simulink model "Propagator"  (R2018a)
settings: Solver=ode4  StartTime=jd_start  StopTime=jd_end  FixedStep=3600  MaxStep=stepsize  RelTol=1e-9  AbsTol=1e-12  EnableMultiTasking=on
values from neighbouring files (symbols this model uses):
  state_ast_initial = [xin; yin; zin; vxin; vyin; vzin]    [driverScript.m]
  state_sat_initial = [xin2; yin2; zin2; vxin2; vyin2; vzin2]    [driverScript.m]
settings Model: Creator=Hridu  LastModifiedBy=Hridu
settings SolverCC: AutoScaleAbsTol=off
settings OptimizationCC: LifeSpan=inf
settings DebuggingCC: SFUnexpectedBacktrackingDiag=warning  SFNoUnconditionalDefaultTransitionDiag=warning  SFExecutionAtInitializationDiag=none
settings CodeAppCC: StateflowObjectComments=on
settings GRTTargetCC: TargetLangStandard=C89/C90 (ANSI)  GeneratePreprocessorConditionals=Disable all
settings ConfigComp: CovMetricSettings=dw  CovHtmlReporting=on  CovSaveCumulativeToWorkspaceVar=on  CovSaveSingleToWorkspaceVar=on  CovExternalEMLEnable=off

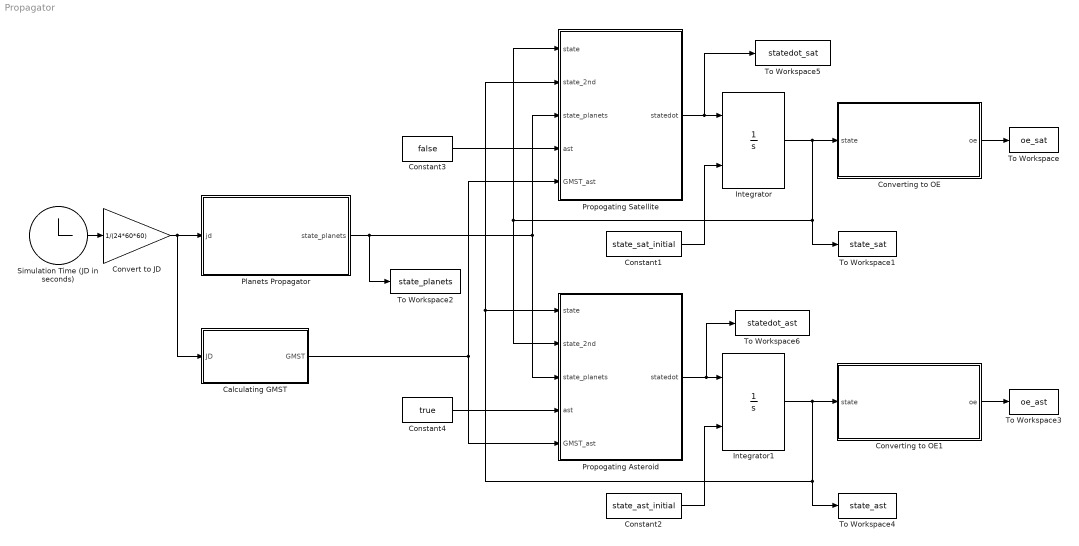
== system Propagator ==
  Calculating GMST : MATLAB Function  TreatAsAtomicUnit=on
  Constant1 : Constant  Value=state_sat_initial
  Constant2 : Constant  Value=state_ast_initial
  Constant3 : Constant  Value=false
  Constant4 : Constant  Value=true
  Convert to JD : Gain  Gain=1/(24*60*60)
  Converting to OE : MATLAB Function  TreatAsAtomicUnit=on
  Converting to OE1 : MATLAB Function  TreatAsAtomicUnit=on
  Integrator : Integrator  InitialConditionSource=external
  Integrator1 : Integrator  InitialConditionSource=external
  Planets Propagator : MATLAB Function  TreatAsAtomicUnit=on
  Propogating Asteroid : MATLAB Function  TreatAsAtomicUnit=on
  Propogating Satellite : MATLAB Function  TreatAsAtomicUnit=on
  Simulation Time (JD in seconds) : Clock
  To Workspace : ToWorkspace  VariableName=oe_sat  SampleTime=-1
  To Workspace1 : ToWorkspace  VariableName=state_sat  SampleTime=-1
  To Workspace2 : ToWorkspace  VariableName=state_planets  SampleTime=-1
  To Workspace3 : ToWorkspace  VariableName=oe_ast  SampleTime=-1
  To Workspace4 : ToWorkspace  VariableName=state_ast  SampleTime=-1
  To Workspace5 : ToWorkspace  VariableName=statedot_sat  SampleTime=-1
  To Workspace6 : ToWorkspace  VariableName=statedot_ast  SampleTime=-1
  wires:
  Propogating Satellite/1(statedot) -> To Workspace5/1, Integrator/1
  Constant1/1 -> Integrator/2
  Converting to OE/1(oe) -> To Workspace/1
  Simulation Time (JD in seconds)/1 -> Convert to JD/1
  Planets Propagator/1(state_planets) -> To Workspace2/1, Propogating Asteroid/3(state_planets), Propogating Satellite/3(state_planets)
  Integrator/1 -> Propogating Asteroid/2(state_2nd), Propogating Satellite/1(state), To Workspace1/1, Converting to OE/1(state)
  Propogating Asteroid/1(statedot) -> To Workspace6/1, Integrator1/1
  Constant2/1 -> Integrator1/2
  Converting to OE1/1(oe) -> To Workspace3/1
  Integrator1/1 -> Converting to OE1/1(state), Propogating Asteroid/1(state), Propogating Satellite/2(state_2nd), To Workspace4/1
  Constant3/1 -> Propogating Satellite/4(ast)
  Constant4/1 -> Propogating Asteroid/4(ast)
  Calculating GMST/1(GMST) -> Propogating Asteroid/5(GMST_ast), Propogating Satellite/5(GMST_ast)
  Convert to JD/1 -> Calculating GMST/1(JD), Planets Propagator/1(jd)

== matlab function Propagator/Converting to OE ==
  data: state input; oe output
function oe = IJKtoOrbitalElements(state)

oe = zeros(6, 1);

% Position and Velocity
rECI = state(1:3);
vECI = state(4:6);

% Specific Angular Momentum
GM_Earth = 3.986e5;
h = cross(rECI, vECI);
W = h./norm(h);

% Inclination
i = atan2(norm(W(1:2)), W(3));

% Right Ascension of the Ascending Node
Omega = atan2(W(1),-W(2));
if Omega < 0
    Omega = Omega + 2*pi;
end

% Semi-Major Axis
a = (2/norm(rECI) - norm(vECI)^2/GM_Earth)^-1;

% Eccentricity
p = norm(h)^2/GM_Earth;
e = sqrt(1 - p/a);

% True Anomaly
n = sqrt(GM_Earth/a^3);
E = atan2((dot(rECI, vECI)/(n*a^2)), (1 - norm(rECI)/a));
if E < 0
    E = E + 2*pi;
end

nu = atan2(a*sqrt(1-e^2)*sin(E),a*(cos(E)-e));
if nu < 0
    nu = nu + 2*pi;
end

% Argument of Periapsis
u = atan2((rECI(3)/sin(i)), (rECI(1)*cos(Omega) + rECI(2)*sin(Omega)));
if u < 0
    u = u + 2*pi;
end

omega = u - nu;
if omega < 0
    omega = omega + 2*pi;
end

oe(1) = a;
oe(2) = e;
oe(3) = i;
oe(4) = Omega;
oe(5) = omega;
oe(6) = nu;

end

== matlab function Propagator/Propogating Satellite ==
  data: state input; state_2nd input; statedot output; state_planets input; ast input; GMST_ast input
function statedot = f(state, state_2nd, state_planets, ast, GMST_ast)

X = load('constants.mat');
statedot = zeros(6, 1);

% Solar Radiation Pressure
if ast == false
    f_srp = accelSRP(state, X.state_sun, state_2nd, X.R_ast,...
        X.Csrp_sat, X.Msrp_sat, X.Asrp_sat, X.Psrp);
else
    f_srp = accelSRP(state, X.state_sun, state_2nd, 0,...
        X.Csrp_ast, X.Msrp_ast, X.Asrp_ast, X.Psrp);
end

% Drag
%f_drag = accelDrag(state);

% Asteroid Gravity
if ast == false
    f_2nd = accelHarmonic(state, state_2nd, X.GM_ast, X.R_ast, GMST_ast);
else
    f_2nd = accelPointMass(state, state_2nd, X.GM_sat);
end

% Sun Gravity
f_sun = X.GM_Sun*state(1:3)/(norm(state(1:3))^3);

% Planets Gravity
f_planets = zeros(3, 1);
for planetid = 1:9
    f_planets = f_planets + accelPointMass(state, state_planets(planetid, :)', X.GM_Planets(planetid));
end

% Calculating StateDot
statedot(1:3) = state(4:6);
statedot(4:6) = -1*(f_2nd + f_sun);% + f_planets);
%statedot(4:6) = -1*f_sun;
end

== matlab function Propagator/Planets Propagator ==
  data: jd input; state_planets output
function state_planets = statePlanetsUnpertubed(jd)
state_planets = zeros(9, 6);
for planet_id = 1:9
    [r, v] = AA279planet_state(planet_id, jd);
    state_planets(planet_id, :) = [r', v'];
end
end

function [O_r_P__heli, heli_v_P__heli] = AA279planet_state(planet_id, jd)
% Returns heliocentric position and velocity of planet at given time
%
% AA279 Function Library
% Last modified: 22 April 2016 by Andrew K. Barrows

% Physical constants from http://ssd.jpl.nasa.gov/horizons.cgi  Feb 2014
km_per_au = 149597870.700; % [km/AU]
musun     = 1.3271244004193938e11; % [km^3/sec^2]

% Get data for selected planet
[j2000_elements, rates] = AA279j2000_planetary_elements(planet_id);

% Find elements at given time
elements = j2000_elements + rates*(jd - 2451545)/36525;

a = elements(1)*km_per_au; % semi-major axis
ecc = elements(2); % eccentricity

p = a*(1 - ecc*ecc); % [km]

inc = elements(3); % [deg] inclination (assume stays in [-90 +90] range)

LAN = elements(4); % [deg] longitude of ascending node
while LAN >= 360.0
    LAN = LAN - 360.0; 
end
while LAN < 0.0
    LAN = LAN + 360.0;
end

omega_bar = elements(5); % [deg] longitude of perihelion
while omega_bar >= 360.0
    omega_bar = omega_bar - 360.0; 
end
while omega_bar < 0.0
    omega_bar = omega_bar + 360.0;
end

L = elements(6); % [deg] mean longitude
while L >= 360.0
    L = L - 360.0; 
end
while L < 0.0
    L = L + 360.0;
end  

omega = omega_bar - LAN; % [deg] argument of perihelion
while omega >= 360.0
    omega = omega - 360.0; 
end
while omega < 0.0
    omega = omega + 360.0;
end 

M = L - omega_bar; % [deg] mean anomaly
while M >= 360.0
    M = M - 360.0; 
end
while M < 0.0
    M = M + 360.0;
end 

% Find eccentric anomaly by solving Kepler's equation
E = AA279solve_kepler(M*pi/180, ecc, 1e-10); % [rad]

% Find position and velocity of planet in perifocal coordinates
sinnu = (sin(E)*sqrt(1.0-ecc*ecc))/(1.0-ecc*cos(E));
cosnu = (cos(E)-ecc)/(1.0-ecc*cos(E));
r = p/(1.0+ecc*cosnu); % Trajectory Equation
O_r_P__peri = [r*cosnu; r*sinnu; 0.0];
sqrtmuoverp = sqrt(musun/p);
peri_v_P__peri = [-sqrtmuoverp*sinnu; sqrtmuoverp*(ecc+cosnu); 0.0];
      
% Convert perifocal coordinates to heliocentric coordinates
sinLAN = sin(LAN*pi/180.0);
cosLAN = cos(LAN*pi/180.0);
sininc = sin(inc*pi/180.0);
cosinc = cos(inc*pi/180.0);
sinomega = sin(omega*pi/180.0);
cosomega = cos(omega*pi/180.0);
heli_C_peri = [+cosLAN*cosomega-sinLAN*sinomega*cosinc ...
                  -cosLAN*sinomega-sinLAN*cosomega*cosinc ...
                      +sinLAN*sininc; ...
              +sinLAN*cosomega+cosLAN*sinomega*cosinc ...
                  -sinLAN*sinomega+cosLAN*cosomega*cosinc ...
                      -cosLAN*sininc; ...       
              +sinomega*sininc ...
                  +cosomega*sininc ...
                      +cosinc];
O_r_P__heli = heli_C_peri*O_r_P__peri;
heli_v_P__heli = heli_C_peri*peri_v_P__peri; % because heli_omega_peri = 0

end % terminates MATLAB function


function [E] = AA279solve_kepler(M, e, tol)
% Solves Kepler's Equation using Newton's method
%
% AA279 Function Library
% Last modified: 22 April 2016 by Andrew K. Barrows
%
% E    Eccentric Anomaly [rad]
% M    Mean Anomaly [rad]
% e    eccentricity [dimensionless]
% tol  tolerance value on E for stopping iteration [rad]

E   = (pi+M)/2;  % initial guess
err = tol + 1.0; % ensures at least one iteration will take place

% Iterate using Newton's method
while err >= tol
    Enew = E + (M-E+e*sin(E))/(1-e*cos(E));
    err = abs(Enew-E);
    E = Enew;
end

end % terminates MATLAB function

function [elements, rates] = AA279j2000_planetary_elements(planet_id)
% Returns a planet's J2000 orbital elements and centennial rates
%
% AA279 Function Library
% Last modified: 22 April 2016 by Andrew K. Barrows
%
% Adapted from Orbital Mechanics for Engineering Students by Howard Curtis
% 
% Data valid for the period 1800 AD - 2050 AD
% Source of data: http://ssd.jpl.nasa.gov/?planet_pos
%
% planet_id: 1 through 9, for Mercury through Pluto
%  
% elements:  row vector of J2000 orbital elements for "planet_id"
%                a             semimajor axis [AU]
%                e             eccentricity
%                i             inclination [deg]
%                OMEGA         longitude of the ascending node [deg]
%                omega_bar     longitude of perihelion [deg]
%                L             mean longitude [deg]                   
%                                         
% rates:     row vector of J2000 centennial rates for "planet_id"    
%                a_dot         [AU/cty] (AU per century)
%                e_dot         [1/cty]
%                i_dot         [deg/cty]
%                OMEGA_dot     [deg/cty]
%                omega_bar_dot [deg/cty]
%                L_dot         [deg/cty]
%
%     a           e          i          OMEGA      omega_bar        L

J2000_elements = ...
[0.38709927  0.20563593  7.00497902  48.33076593  77.45779628  252.25032350
 0.72333566  0.00677672  3.39467605  76.67984255 131.60246718  181.97909950 
 1.00000261  0.01671123 -0.00001531   0.0        102.93768193  100.46457166 
 1.52371034  0.09339410  1.84969142  49.55953891 -23.94362959 	-4.55343205
 5.20288700  0.04838624  1.30439695 100.47390909  14.72847983 	34.39644501
 9.53667594  0.05386179  2.48599187 113.66242448  92.59887831 	49.95424423
19.18916464  0.04725744  0.77263783  74.01692503 170.95427630  313.23810451
30.06992276  0.00859048  1.77004347 131.78422574  44.96476227  -55.12002969 
39.48211675  0.24882730 17.14001206 110.30393684 224.06891629  238.92903833];

centennial_rates = ... 
[0.00000037  0.00001906 -0.00594749 -0.12534081  0.16047689  149472.67411175 
 0.00000390 -0.00004107 -0.00078890 -0.27769418  0.00268329	  58517.81538729  
 0.00000562 -0.00004392 -0.01294668  0.0         0.32327364   35999.37244981  
 0.0001847 	 0.00007882 -0.00813131 -0.29257343  0.44441088   19140.30268499  
-0.00011607 -0.00013253 -0.00183714  0.20469106	 0.21252668    3034.74612775 
-0.00125060 -0.00050991  0.00193609 -0.28867794 -0.41897216    1222.49362201
-0.00196176 -0.00004397 -0.00242939  0.04240589  0.40805281 	428.48202785 
 0.00026291  0.00005105  0.00035372 -0.00508664 -0.32241464 	218.45945325 
-0.00031596  0.00005170  0.00004818 -0.01183482 -0.04062942 	145.20780515]; 
 
elements = J2000_elements(planet_id, :);
rates = centennial_rates(planet_id, :);
end % terminates MATLAB function

== matlab function Propagator/Converting to OE1 ==
  data: state input; oe output
function oe = IJKtoOrbitalElements(state)

oe = zeros(6, 1);

% Position and Velocity
rECI = state(1:3);
vECI = state(4:6);

% Specific Angular Momentum
GM_Sun = 1.327124400179870e11;
h = cross(rECI, vECI);
W = h./norm(h);

% Inclination
i = atan2(norm(W(1:2)), W(3));

% Right Ascension of the Ascending Node
Omega = atan2(W(1),-W(2));
if Omega < 0
    Omega = Omega + 2*pi;
end

% Semi-Major Axis
a = (2/norm(rECI) - norm(vECI)^2/GM_Sun)^-1;

% Eccentricity
p = norm(h)^2/GM_Sun;
e = sqrt(1 - p/a);

% True Anomaly
n = sqrt(GM_Sun/a^3);
E = atan2((dot(rECI, vECI)/(n*a^2)), (1 - norm(rECI)/a));
if E < 0
    E = E + 2*pi;
end

nu = atan2(a*sqrt(1-e^2)*sin(E),a*(cos(E)-e));
if nu < 0
    nu = nu + 2*pi;
end

% Argument of Periapsis
u = atan2((rECI(3)/sin(i)), (rECI(1)*cos(Omega) + rECI(2)*sin(Omega)));
if u < 0
    u = u + 2*pi;
end

omega = u - nu;
if omega < 0
    omega = omega + 2*pi;
end

oe(1) = a;
oe(2) = e;
oe(3) = i;
oe(4) = Omega;
oe(5) = omega;
oe(6) = nu;

end

== matlab function Propagator/Propogating Asteroid ==
  data: state input; state_2nd input; statedot output; state_planets input; ast input; GMST_ast input
function statedot = f(state, state_2nd, state_planets, ast, GMST_ast)

X = load('constants.mat');
statedot = zeros(6, 1);

% Solar Radiation Pressure
if ast == false
    f_srp = accelSRP(state, X.state_sun, state_2nd, X.R_ast,...
        X.Csrp_sat, X.Msrp_sat, X.Asrp_sat, X.Psrp);
else
    f_srp = accelSRP(state, X.state_sun, state_2nd, 0,...
        X.Csrp_ast, X.Msrp_ast, X.Asrp_ast, X.Psrp);
end

% Drag
%f_drag = accelDrag(state);

% Asteroid Gravity
if ast == false
    f_2nd = accelHarmonic(state, state_2nd, X.GM_ast, X.R_ast, GMST_ast);
else
    f_2nd = accelPointMass(state, state_2nd, X.GM_sat);
end

% Sun Gravity
f_sun = X.GM_Sun*state(1:3)/(norm(state(1:3))^3);

% Planets Gravity
f_planets = zeros(3, 1);
for planetid = 1:9
    f_planets = f_planets + accelPointMass(state, state_planets(planetid, :)', X.GM_Planets(planetid));
end

% Calculating StateDot
statedot(1:3) = state(4:6);
statedot(4:6) = -1*(f_2nd + f_sun);% + f_planets);
%statedot(4:6) = -1*f_sun;
end

== matlab function Propagator/Calculating GMST ==
  data: JD input; GMST output
function GMST  = JDtoGMST(JD)
MJD = JD - 2400000.5;
d = MJD - 51544.5;

GMST = 1639.46869*d;
%Earth
%GMST = 280.4606 + 360.9856473*d;
GMST = mod(GMST, 360);
end
